simulink model "OneTwo_allBlock"  (R2022b)
settings: Solver=VariableStepAuto  StartTime=0.0  StopTime=1  RelTol=1e-3
settings Model: Creator=yeyi5  LastModifiedBy=yeyi5

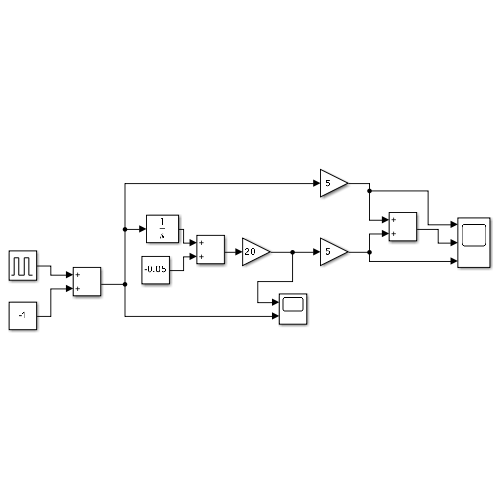
[thumbnail: Simulink's stored preview of the top-level diagram]
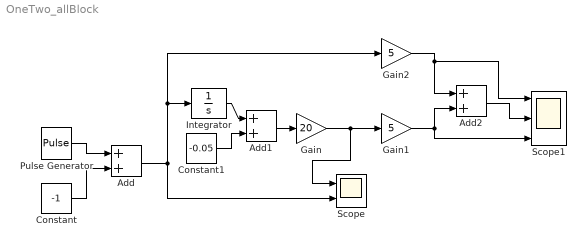
== system OneTwo_allBlock ==
  Add : Sum
  Add1 : Sum
  Add2 : Sum
  Constant : Constant  Value=-1
  Constant1 : Constant  Value=-0.05
  Gain : Gain  Gain=20
  Gain1 : Gain  Gain=5
  Gain2 : Gain  Gain=5
  Integrator : Integrator
  Pulse Generator : DiscretePulseGenerator  PulseType=Time based  Amplitude=2  Period=1/5  PulseWidth=50
  Scope : Scope  NumInputPorts=2
  Scope1 : Scope  NumInputPorts=3
  wires:
  Pulse Generator/1 -> Add/1
  Constant/1 -> Add/2
  Add/1 -> Scope/2, Gain2/1, Integrator/1
  Integrator/1 -> Add1/1
  Constant1/1 -> Add1/2
  Add1/1 -> Gain/1
  Gain/1 -> Gain1/1, Scope/1
  Gain1/1 -> Add2/2, Scope1/3
  Add2/1 -> Scope1/2
  Gain2/1 -> Scope1/1, Add2/1
